simulink model "sgMdl_IO132_DMALoopback"  (R2024b)
settings: Solver=FixedStepAuto  StartTime=0.0  StopTime=inf  RelTol=1e-3  EnableMultiTasking=on
libraries: speedgoatlib_IO132 x3, speedgoatlib_interrupt x1, dspsrcs4 x1
Description:
  | IO132 - DMA Loopback
settings Model: sg_rtwmakecfg_data=_sglibc_  ModifiedByFormat=Speedgoat  Creator=Speedgoat  LastModifiedBy=Speedgoat
settings SolverCC: ConcurrentTasks=on  AlgebraicLoopSolver=TrustRegion  PositivePriorityOrder=on  AutoInsertRateTranBlk=on  InsertRTBMode=Never (minimum delay)
settings DataIOCC: SaveFormat=StructureWithTime  ReturnWorkspaceOutputs=off
settings OptimizationCC: BlockReduction=off  OptimizeBlockIOStorage=off  BufferReuse=off  GlobalBufferReuse=off  ExpressionFolding=off  LocalBlockOutputs=off
settings DebuggingCC: TasksWithSamePriorityMsg=none  UnconnectedInputMsg=warning  UnconnectedOutputMsg=warning  UnconnectedLineMsg=warning  SFExecutionAtInitializationDiag=none  ArithmeticOperatorsInVariantConditions=warning
settings HardwareCC: ProdBitPerLong=64  ProdLongLongMode=on  ProdHWDeviceType=Intel->x86-64 (Linux 64)
settings ModelReferenceCC: EnableRefExpFcnMdlSchedulingChecks=on
settings SFSimCC: SimUseLocalCustomCode=off  CustomCodeUndefinedFunction=UseInterfaceOnly
settings RTWCC: Description=Speedgoat Real-Time Target Machine  SystemTargetFile=speedgoat.tlc  TemplateMakefile=slrealtime_default_tmf  RTWUseLocalCustomCode=off  Toolchain=Simulink Real-Time Toolchain  BuildConfiguration=Faster Runs  TargetLang=C++  GPUComputeCapability=3.5  DLArmComputeVersion=19.05
settings CodeAppCC: StateflowObjectComments=on
settings SimulinkRealTimeTargetCC: SubcomponentCodeInterfacePackaging=Reusable function  InstructionSetFMA=off  LogToMDFFile=off  SLRTFileLogMaxRuns=10  UseGCCFastMath=on
settings ConfigComp: CovBoundaryAbsTol=1.0e-5

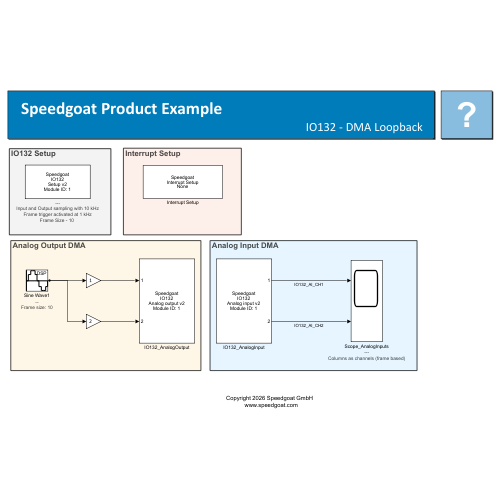
[thumbnail: Simulink's stored preview of the top-level diagram]
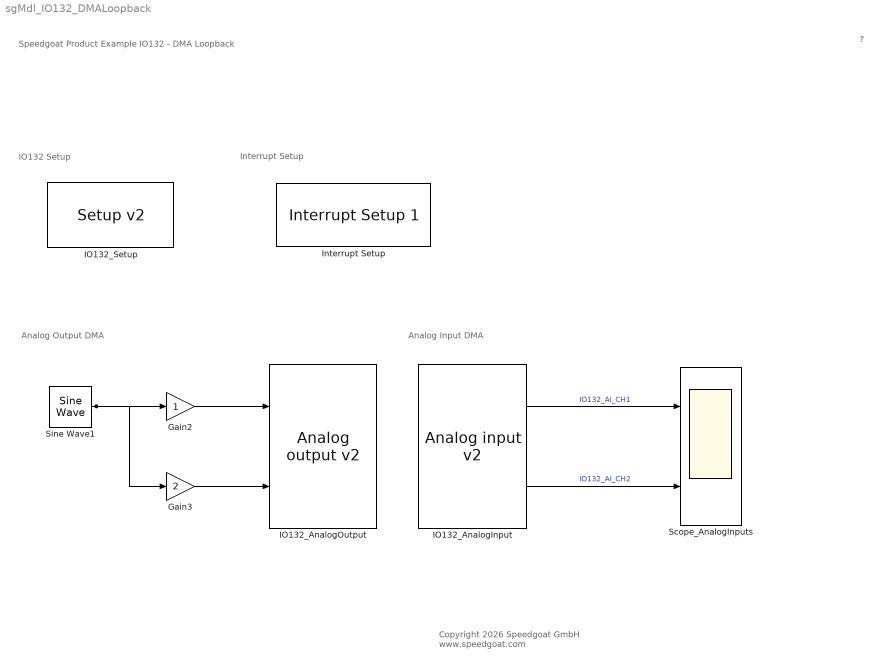
== system sgMdl_IO132_DMALoopback ==
  note: Interrupt Setup
  note: IO132 Setup
  note: Analog Input DMA
  note: Analog Output DMA
  note: Speedgoat Product Example
      | IO132 - DMA Loopback
  note: ?
  note: Copyright 2026 Speedgoat GmbH
      |  www.speedgoat.com
  Gain2 : Gain
  Gain3 : Gain  Gain=2
  IO132_AnalogInput : speedgoatlib_IO132/Analog input v2   parModuleId=1  parSampleTime=-1  parPciSlot=-1  parAdcChannels=[1 2]  parAdcVoltageRange=2  parAdcOversamplRate=1  parAdcContSampling=0  parAdcDmaEnable=1  parAdcActiveDmaDevices=1  parAdcFrameSize=10
      settings: SourceProductName=Simulink Real-Time: Speedgoat I/O Driver Library
  IO132_AnalogOutput : speedgoatlib_IO132/Analog output v2   parModuleId=1  parSampleTime=-1  parPciSlot=-1  parDacChannels=[1 2]  parDacVoltageRange=[5 5 5 5]  parDacInitValues=[0 0]  parDacReset=[1 1]  parDacSyncOut=1  parDacDmaEnable=1  parDacActiveDmaDevices=1  parDacDmaLatency=2  parDacFrameSize=10
      settings: SourceProductName=Simulink Real-Time: Speedgoat I/O Driver Library
  IO132_Setup : speedgoatlib_IO132/Setup v2   parPciSlot=-1  parModuleId=1  parInterModuleSync=None  parConvClockBaseRate=20MHz  parConvClock1Divider=2000  parConvClock2Divider=2000  parFrameTriggerEnable=on  parFrameTriggerDivider=10  parConvClock1BaseRate=1  parConvClock2BaseRate=1  parFrameTriggerClock=1  parAdcChannels=[1 2]  parAdcRange1=+-10V  parAdcVoltageRange=2  parAdcOversampling1=None  parAdcOversamplRate=1  parAdcContSampling=off  parAdcDataCorrection=Automatic  parAdcCorrectionActive={}  parAdcCorrectionPm5V={'1','0','0';'2','0','0';'3','0','0';'4','0','0';'5','0','0';'6','0','0';'7','0','0';'8','0','0'}  parAdcCorrectionPm10V={'1','0','0';'2','0','0';'3','0','0';'4','0','0';'5','0','0';'6','0','0';'7','0','0';'8','0','0'}  parAdcDmaEnable=on  parAdcDmaClock=Clock 1  parAdcFrameSize_=10  parAdcSampleTime_=-1  parAdcActiveDmaDevices=[1]  parAdcFrameTriggerEnable=1  parAdcFrameSize=10  parAdcSampleTime=0.001  parDacChannels=[1 2]  parDacInitValues=0  parDacReset=1  parDacRange1=+-10V  parDacRange2=+-10V  parDacRange3=+-10V  parDacRange4=+-10V  parDacVoltageRange=[5 5 5 5]  parDacSyncOut=on  parDacDataCorrection=Automatic  parDacCorrectionActive={}  parDacCorrection5V={'1','0','0';'2','0','0';'3','0','0';'4','0','0'}  parDacCorrection10V={'1','0','0';'2','0','0';'3','0','0';'4','0','0'}  parDacCorrection10_8V={'1','0','0';'2','0','0';'3','0','0';'4','0','0'}  parDacCorrectionPm5V={'1','0','0';'2','0','0';'3','0','0';'4','0','0'}  parDacCorrectionPm10V={'1','0','0';'2','0','0';'3','0','0';'4','0','0'}  parDacCorrectionPm10_8V={'1','0','0';'2','0','0';'3','0','0';'4','0','0'}  parDacDmaEnable=on  parDacDmaLatency=Until next frame  parDacDmaClock=Clock 1  parDacFrameSize_=10  parDacSampleTime_=-1  parDacActiveDmaDevices=[1]  parDacFrameTriggerEnable=1  parDacFrameSize=10  parDacSampleTime=0.001  parDoChannels=[1]  parDoInitValues=0  parDoReset=1  parDiChannels=[5]  parDiDebounceEnable=off  parDiDebounceTime=0  parDiDebounceValue=0  parDioPullRefFront=Pull-up 3.3V  parDioPullRefRear=Floating
      settings: SourceProductName=Simulink Real-Time: Speedgoat I/O Driver Library
      settings: AttributesFormatString=|
      | ---
      | Input and Output sampling with 10 kHz
      | Frame trigger activated at 1 kHz
      | Frame Size - 10
  Interrupt Setup : speedgoatlib_interrupt/Interrupt Setup 1  parModuleTrigger=on  parPollingMode=off  parPriorityConf=High  parPriority=241  confStartFcn=IO132_start_public  confStopFcn=IO132_stop_public  confIsrFcn=IO132_isr_public  confMapFcn=IO132_map_public  confHookFile=io132_int_hooks.c  confIrqNr=-1  confIsPolling=off  confModID=16776961  confSelectedInt=Speedgoat IO132 DMA interrupt  confSelectedId=1  confSelectedChannel=[]  confData=[]  confForcePollingMode=off
  Scope_AnalogInputs : Scope  NumInputPorts=2
      settings: AttributesFormatString=|
      | ---
      | %<FrameBasedProcessingString>
  Sine Wave1 : dspsrcs4/Sine Wave  Amplitude=1  Frequency=100  Phase=0  SampleMode=Discrete  OutComplex=Real  CompMethod=Trigonometric fcn  TableSize=Speed  SampleTime=1/10000  SamplesPerFrame=10  ResetState=Restart at time zero  OutputFrames=off  dataType=double  wordLen=16  udDataType=sfix(16)  fracBitsMode=Best precision  numFracBits=15  OutDataTypeStr=double  LastOutDataTypeStr=double
      settings: AttributesFormatString=|
      | --
      | Frame size: %<SamplesPerFrame>
  wires:
  IO132_AnalogInput/1 -> Scope_AnalogInputs/1  "IO132_AI_CH1"
  Gain2/1 -> IO132_AnalogOutput/1
  Gain3/1 -> IO132_AnalogOutput/2
  IO132_AnalogInput/2 -> Scope_AnalogInputs/2  "IO132_AI_CH2"
  Sine Wave1/1 -> Gain2/1, Gain3/1
